simulink model "impluseModel"  (R2019b)
settings: Solver=ode8  StartTime=0.0  StopTime=86400  FixedStep=60  RelTol=1e-3
values from neighbouring files (symbols this model uses):
  r0 = zeros(3,2)    [primeVectorAnalyze.m]
undefined symbols (not defined in the file or in its folder): v0
settings Model: Creator=yanhuida  LastModifiedBy=yanhuida

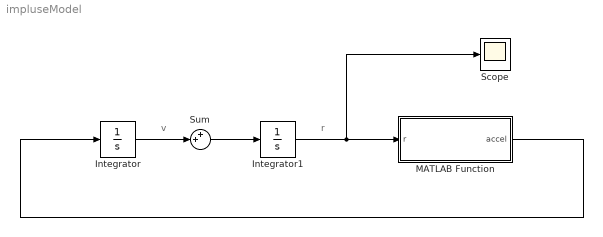
== system impluseModel ==
  note: v
  note: r
  Integrator : Integrator  InitialCondition=v0
  Integrator1 : Integrator  InitialCondition=r0
  MATLAB Function : MATLAB Function  TreatAsAtomicUnit=on
  Scope : Scope
  Sum : Sum  Inputs=++|
  wires:
  MATLAB Function/1(accel) -> Integrator/1
  Integrator1/1 -> Scope/1, MATLAB Function/1(r)
  Integrator/1 -> Sum/2
  Sum/1 -> Integrator1/1

== matlab function impluseModel/MATLAB Function ==
  data: accel output size=[3 1]; r input size=[3 1]
function accel = TwoBodyModel(r)
GM_Earth = 3.986004415e5;
accel = -GM_Earth / (r(1)^2 + r(2)^2 + r(3)^2)^(1.5) * r;
end
